simulink model "cic_dezim2_"  (Simulink 7.8)
settings: Solver=FixedStepDiscrete  StartTime=0.0  StopTime=1  RelTol=1e-3
undefined symbols (not defined in the file or in its folder): cfir
libraries: dspsigops x8, dspsrcs4 x1
settings Model: Creator=svenhoffmann  LastModifiedBy=josef  ExtModeAutoUpdateStatusClock=off
settings OptimizationCC: InlineInvariantSignals=on  InitFltsAndDblsToZero=on
settings DebuggingCC: SaveWithParameterizedLinksMsg=none  SignalResolutionControl=TryResolveAllWithWarning  MultiTaskDSMMsg=warning  MultiTaskCondExecSysMsg=none  FcnCallInpInsideContextMsg=Use local settings  StrictBusMsg=None
settings RTWCC: IncludeERTFirstTime=on
settings GRTTargetCC: TargetFcnLib=ansi_tfl_tmw.mat

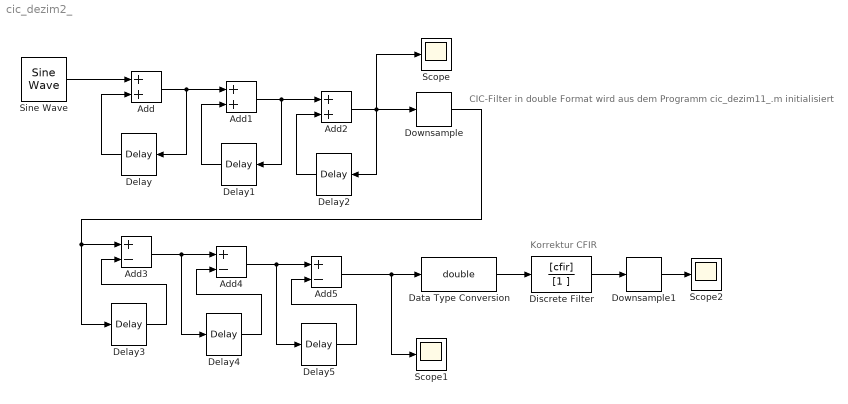
== system cic_dezim2_ ==
  note: Korrektur CFIR
  note: CIC-Filter
      | in double
      | Format
      | wird aus dem Programm
      | cic_dezim11_.m
      | initialisiert
  Add : Sum
  Add1 : Sum
  Add2 : Sum
  Add3 : Sum  Inputs=+-
  Add4 : Sum  Inputs=+-
  Add5 : Sum  Inputs=+-
  Data Type Conversion : DataTypeConversion  OutDataTypeStr=double
  Delay{,1..5} (6 alike) : dspsigops/Delay  InputProcessing=Inherited (this choice will be removed - see release notes)  dly_unit=Samples  delay=1  ic_detail=off  dif_ic_for_ch=off  dif_ic_for_dly=off  ic=0  reset_popup=None
  Discrete Filter : DiscreteFilter  Numerator=[cfir]  Denominator=[1 ]
  Downsample : dspsigops/Downsample  N=5  phase=0  InputProcessing=Inherited (this choice will be removed - see release notes)  RateOptions=Enforce single-rate processing  smode=Allow multirate  fmode=Maintain input frame size  ic=0
  Downsample1 : dspsigops/Downsample  N=2  phase=0  InputProcessing=Inherited (this choice will be removed - see release notes)  RateOptions=Enforce single-rate processing  smode=Allow multirate  fmode=Maintain input frame size  ic=0
  Scope : Scope
  Scope1 : Scope
  Scope2 : Scope
      settings: YMin=-100  YMax=100  SaveName=ScopeData2
  Sine Wave : dspsrcs4/Sine Wave  Amplitude=0.75  Frequency=10000/(fix(10000/10))  Phase=0  SampleMode=Discrete  OutComplex=Real  CompMethod=Table lookup  TableSize=Speed  SampleTime=1/10000  SamplesPerFrame=1  ResetState=Restart at time zero  dataType=double  wordLen=16  udDataType=sfix(16)  fracBitsMode=User-defined  numFracBits=8  OutDataTypeStr=double  LastOutDataTypeStr=double
  wires:
  Sine Wave/1 -> Add/1
  Delay/1 -> Add/2
  Add/1 -> Delay/1, Add1/1
  Delay1/1 -> Add1/2
  Add1/1 -> Delay1/1, Add2/1
  Add2/1 -> Delay2/1, Scope/1, Downsample/1
  Delay2/1 -> Add2/2
  Delay3/1 -> Add3/2
  Delay4/1 -> Add4/2
  Delay5/1 -> Add5/2
  Add3/1 -> Add4/1, Delay4/1
  Add4/1 -> Add5/1, Delay5/1
  Downsample/1 -> Add3/1, Delay3/1
  Add5/1 -> Scope1/1, Data Type Conversion/1
  Data Type Conversion/1 -> Discrete Filter/1
  Discrete Filter/1 -> Downsample1/1
  Downsample1/1 -> Scope2/1
